simulink model "threeTetherVerification_th"  (R2018b)
settings: Solver=ode15s  StartTime=0.0  StopTime=duration_s  MaxStep=5  RelTol=1e-3  AbsTol=1e-3
undefined symbols (not defined in the file or in its folder): ayazPlant, ayazPlant_cl, gnd_station, ini_euler_ang, ini_Rcm_o, R11_g, R1n_cm, R21_g, R2n_cm, R31_g, R3n_cm, rotation_sequence, sim_param, Subsystem1, threeTethers_cl
libraries: singleTether_cl x3, ayazController_cl x1, ayazFlow_cl x1, ayazLiftingBody_cl x1, ayazWinches_cl x1, threeTetherGroundStation_cl x1
settings Model: Creator=mcobb  LastModifiedBy=mcobb

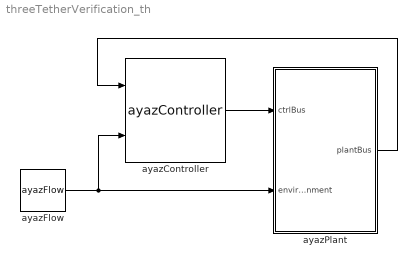
== system threeTetherVerification_th ==
  ayazController : ayazController_cl/ayazController  SystemSampleTime=-1  VariantControl=VSS_controller_ayazController
  ayazFlow : ayazFlow_cl/ayazFlow  SystemSampleTime=-1
  ayazPlant : Subsystem  AncestorBlock=ayazPlant_cl/ayazPlant
  wires:
  ayazController/1 -> ayazPlant/1(ctrlBus)
  ayazPlant/1(plantBus) -> ayazController/1
  ayazFlow/1 -> ayazController/2, ayazPlant/2(environment)

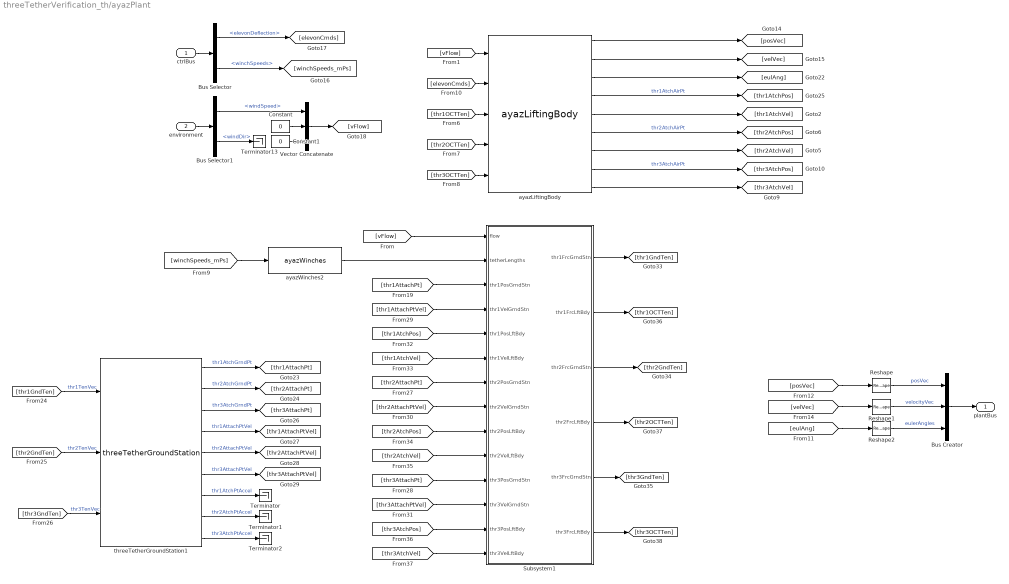
== system threeTetherVerification_th/ayazPlant ==
  ctrlBus : Inport  OutDataTypeStr=Bus: ctrlBus
  environment : Inport  Port=2  OutDataTypeStr=Bus: envBus
  Bus Creator : BusCreator  Inputs=3  OutDataTypeStr=Bus: plantBus
  Bus Selector : BusSelector  OutputSignals=elevonDeflection,winchSpeeds
  Bus Selector1 : BusSelector  OutputSignals=windSpeed,windDir
  Constant : Constant  Value=0
  Constant1 : Constant  Value=0
  Reshape : Reshape  OutputDimensionality=Column vector (2-D)
  Reshape1 : Reshape  OutputDimensionality=Column vector (2-D)
  Reshape2 : Reshape  OutputDimensionality=Column vector (2-D)
  Subsystem1 : Subsystem  AncestorBlock=threeTethers_cl/Subsystem1
  Terminator{,1..2,13} (4 alike) : Terminator
  Vector Concatenate : Concatenate  NumInputs=3
  ayazLiftingBody : ayazLiftingBody_cl/ayazLiftingBody  SystemSampleTime=-1
  ayazWinches2 : ayazWinches_cl/ayazWinches  maxSpeed=maxWinchSpeed  maxAccel=maxWinchAccel  timeConst=1  tetherLengths=unstretched_l
  threeTetherGroundStation1 : threeTetherGroundStation_cl/threeTetherGroundStation  fixed=1  J=sim_param.platform_param.platform_Izz  b=sim_param.platform_param.platform_damping  posVec=[0 0 0]  thr1AttachPt=sim_param.tether_imp_nodes.R11_g  thr2AttachPt=sim_param.tether_imp_nodes.R21_g  thr3AttachPt=sim_param.tether_imp_nodes.R31_g  initAngPos=ini_platform_ang  initAngVel=ini_platform_vel
  plantBus : Outport  OutDataTypeStr=Bus: plantBus
  wires:
  [eulAng] -> Reshape2/1
  [velVec] -> Reshape1/1
  [posVec] -> Reshape/1
  Subsystem1/5(thr3FrcGrndStn) -> [thr3GndTen]
  Subsystem1/6(thr3FrcLftBdy) -> [thr3OCTTen]
  Subsystem1/4(thr2FrcLftBdy) -> [thr2OCTTen]
  Subsystem1/3(thr2FrcGrndStn) -> [thr2GndTen]
  Subsystem1/2(thr1FrcLftBdy) -> [thr1OCTTen]
  Subsystem1/1(thr1FrcGrndStn) -> [thr1GndTen]
  [thr1AtchVel] -> Subsystem1/6(thr1VelLftBdy)
  [thr2AtchPos] -> Subsystem1/9(thr2PosLftBdy)
  [thr2AtchVel] -> Subsystem1/10(thr2VelLftBdy)
  [thr3AtchPos] -> Subsystem1/13(thr3PosLftBdy)
  [thr3AtchVel] -> Subsystem1/14(thr3VelLftBdy)
  [thr1AtchPos] -> Subsystem1/5(thr1PosLftBdy)
  [thr1AttachPtVel] -> Subsystem1/4(thr1VelGrndStn)
  [thr2AttachPtVel] -> Subsystem1/8(thr2VelGrndStn)
  [thr3AttachPtVel] -> Subsystem1/12(thr3VelGrndStn)
  [thr3AttachPt] -> Subsystem1/11(thr3PosGrndStn)
  [thr2AttachPt] -> Subsystem1/7(thr2PosGrndStn)
  [thr1AttachPt] -> Subsystem1/3(thr1PosGrndStn)
  [vFlow] -> Subsystem1/1(flow)
  threeTetherGroundStation1/7 -> Terminator/1  "thr1AtchPtAccel"
  [thr1GndTen] -> threeTetherGroundStation1/1  "thr1TenVec"
  [thr3GndTen] -> threeTetherGroundStation1/3  "thr3TenVec"
  [winchSpeeds_mPs] -> ayazWinches2/1
  [thr2GndTen] -> threeTetherGroundStation1/2  "thr2TenVec"
  ayazWinches2/1 -> Subsystem1/2(tetherLengths)
  threeTetherGroundStation1/1 -> [thr1AttachPt]  "thr1AtchGrndPt"
  threeTetherGroundStation1/3 -> [thr3AttachPt]  "thr3AtchGrndPt"
  threeTetherGroundStation1/2 -> [thr2AttachPt]  "thr2AtchGrndPt"
  threeTetherGroundStation1/4 -> [thr1AttachPtVel]  "thr1AttachPtVel"
  threeTetherGroundStation1/8 -> Terminator1/1  "thr2AtchPtAccel"
  threeTetherGroundStation1/5 -> [thr2AttachPtVel]  "thr2AttachPtVel"
  threeTetherGroundStation1/6 -> [thr3AttachPtVel]  "thr3AttachPtVel"
  threeTetherGroundStation1/9 -> Terminator2/1  "thr3AtchPtAccel"
  ayazLiftingBody/9 -> [thr3AtchVel]
  ayazLiftingBody/8 -> [thr3AtchPos]  "thr3AtchAirPt"
  ayazLiftingBody/7 -> [thr2AtchVel]
  ayazLiftingBody/6 -> [thr2AtchPos]  "thr2AtchAirPt"
  ayazLiftingBody/5 -> [thr1AtchVel]
  ayazLiftingBody/4 -> [thr1AtchPos]  "thr1AtchAirPt"
  ayazLiftingBody/3 -> [eulAng]
  Constant1/1 -> Vector Concatenate/3
  Constant/1 -> Vector Concatenate/2
  Vector Concatenate/1 -> [vFlow]
  Reshape1/1 -> Bus Creator/2  "velocityVec"
  Reshape2/1 -> Bus Creator/3  "eulerAngles"
  Reshape/1 -> Bus Creator/1  "posVec"
  Bus Creator/1 -> plantBus/1
  Bus Selector/2 -> [winchSpeeds_mPs]  "<winchSpeeds>"
  Bus Selector1/1 -> Vector Concatenate/1  "<windSpeed>"
  Bus Selector/1 -> [elevonCmds]  "<elevonDeflection>"
  Bus Selector1/2 -> Terminator13/1  "<windDir>"
  ctrlBus/1 -> Bus Selector/1
  environment/1 -> Bus Selector1/1
  [elevonCmds] -> ayazLiftingBody/2
  [thr3OCTTen] -> ayazLiftingBody/5
  [thr2OCTTen] -> ayazLiftingBody/4
  [thr1OCTTen] -> ayazLiftingBody/3
  [vFlow] -> ayazLiftingBody/1
  ayazLiftingBody/2 -> [velVec]
  ayazLiftingBody/1 -> [posVec]

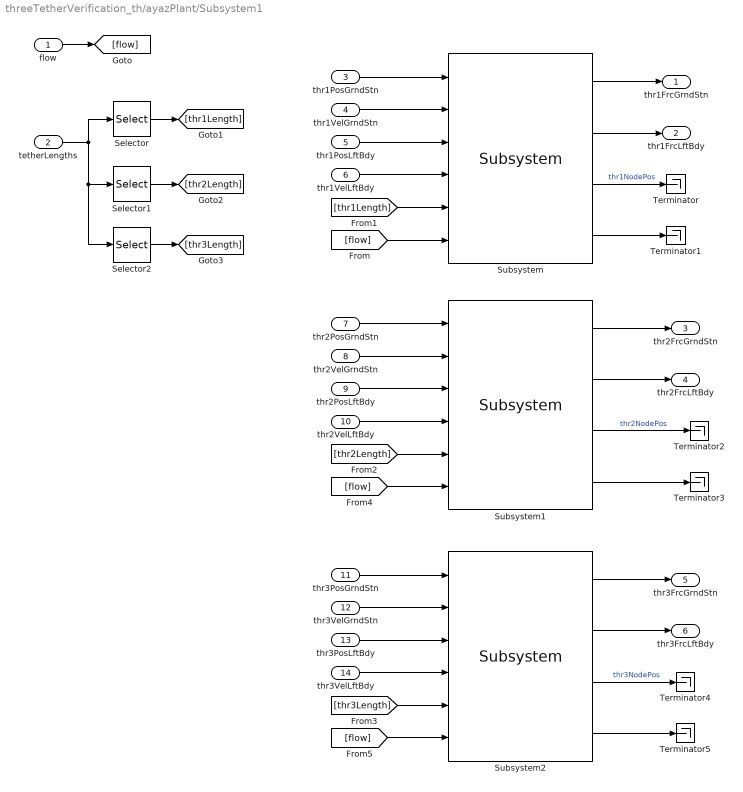
== system threeTetherVerification_th/ayazPlant/Subsystem1 ==
  flow : Inport
  tetherLengths : Inport  Port=2
  thr1PosGrndStn : Inport  Port=3
  thr1VelGrndStn : Inport  Port=4
  thr1PosLftBdy : Inport  Port=5
  thr1VelLftBdy : Inport  Port=6
  thr2PosGrndStn : Inport  Port=7
  thr2VelGrndStn : Inport  Port=8
  thr2PosLftBdy : Inport  Port=9
  thr2VelLftBdy : Inport  Port=10
  thr3PosGrndStn : Inport  Port=11
  thr3VelGrndStn : Inport  Port=12
  thr3PosLftBdy : Inport  Port=13
  thr3VelLftBdy : Inport  Port=14
  Selector : Selector  InputPortWidth=3  IndexOptions=Index vector (dialog)  Indices=1  OutputSizes=1
  Selector1 : Selector  InputPortWidth=3  IndexOptions=Index vector (dialog)  Indices=1  OutputSizes=1
  Selector2 : Selector  InputPortWidth=3  IndexOptions=Index vector (dialog)  Indices=1  OutputSizes=1
  Subsystem : singleTether_cl/Subsystem  N=sim_param.N  dia_t=sim_param.tether_param.tether_diameter(1)  E=sim_param.tether_param.tether_youngs  rho_tether=sim_param.tether_param.tether_density+ sim_param.env_param.density  Cd=sim_param.tether_param.CD_cylinder  zeta=sim_param.tether_param.damping_ratio  rho=sim_param.env_param.density  mass=sim_param.geom_param.mass  ini_Rn_o=ini_Rcm_o + rotation_sequence(ini_euler_ang)*R1n_cm  ini_R1_o=gnd_station + R11_g
  Subsystem1 : singleTether_cl/Subsystem  N=sim_param.N  dia_t=sim_param.tether_param.tether_diameter(2)  E=sim_param.tether_param.tether_youngs  rho_tether=sim_param.tether_param.tether_density+ sim_param.env_param.density  Cd=sim_param.tether_param.CD_cylinder  zeta=sim_param.tether_param.damping_ratio  rho=sim_param.env_param.density  mass=sim_param.geom_param.mass  ini_Rn_o=ini_Rcm_o + rotation_sequence(ini_euler_ang)*R2n_cm  ini_R1_o=gnd_station + R21_g
  Subsystem2 : singleTether_cl/Subsystem  N=sim_param.N  dia_t=sim_param.tether_param.tether_diameter(3)  E=sim_param.tether_param.tether_youngs  rho_tether=sim_param.tether_param.tether_density+ sim_param.env_param.density  Cd=sim_param.tether_param.CD_cylinder  zeta=sim_param.tether_param.damping_ratio  rho=sim_param.env_param.density  mass=sim_param.geom_param.mass  ini_Rn_o=ini_Rcm_o + rotation_sequence(ini_euler_ang)*R3n_cm  ini_R1_o=gnd_station + R31_g
  Terminator{,1..5} (6 alike) : Terminator
  thr1FrcGrndStn : Outport
  thr1FrcLftBdy : Outport  Port=2
  thr2FrcGrndStn : Outport  Port=3
  thr2FrcLftBdy : Outport  Port=4
  thr3FrcGrndStn : Outport  Port=5
  thr3FrcLftBdy : Outport  Port=6
  wires:
  Subsystem1/1 -> thr2FrcGrndStn/1
  Subsystem1/2 -> thr2FrcLftBdy/1
  Subsystem1/3 -> Terminator2/1  "thr2NodePos"
  Subsystem1/4 -> Terminator3/1
  Subsystem2/1 -> thr3FrcGrndStn/1
  Subsystem2/2 -> thr3FrcLftBdy/1
  Subsystem2/3 -> Terminator4/1  "thr3NodePos"
  Subsystem2/4 -> Terminator5/1
  Subsystem/4 -> Terminator1/1
  Subsystem/3 -> Terminator/1  "thr1NodePos"
  Subsystem/2 -> thr1FrcLftBdy/1
  Subsystem/1 -> thr1FrcGrndStn/1
  thr3PosGrndStn/1 -> Subsystem2/1
  thr3VelGrndStn/1 -> Subsystem2/2
  thr3PosLftBdy/1 -> Subsystem2/3
  thr3VelLftBdy/1 -> Subsystem2/4
  thr2VelLftBdy/1 -> Subsystem1/4
  thr2PosLftBdy/1 -> Subsystem1/3
  thr2VelGrndStn/1 -> Subsystem1/2
  thr2PosGrndStn/1 -> Subsystem1/1
  [flow] -> Subsystem2/6
  [flow] -> Subsystem1/6
  [thr3Length] -> Subsystem2/5
  [thr2Length] -> Subsystem1/5
  [thr1Length] -> Subsystem/5
  Selector2/1 -> [thr3Length]
  Selector1/1 -> [thr2Length]
  tetherLengths/1 -> Selector2/1, Selector1/1, Selector/1
  Selector/1 -> [thr1Length]
  [flow] -> Subsystem/6
  flow/1 -> [flow]
  thr1PosLftBdy/1 -> Subsystem/3
  thr1VelLftBdy/1 -> Subsystem/4
  thr1VelGrndStn/1 -> Subsystem/2
  thr1PosGrndStn/1 -> Subsystem/1
